simulink model "test_kalman_paper"  (R2023b)
settings: Solver=VariableStepAuto  StartTime=0.0  StopTime=30  RelTol=1e-3
values from neighbouring files (symbols this model uses):
  P0 = diag([0.01, 0.01, 0.01, 0.01, 0.01, 0.01])    [initialize_paper.m]
  Sigma = diag([0.05, 0.05, 0.05, 0.00001, 0.00001, 0.00001])    [initialize_paper.m]
  Theta = diag([0.05,0.05,0.05])    [initialize_paper.m]
libraries: simulink x2
settings Model: Creator=joaolehodey  LastModifiedBy=joaolehodey

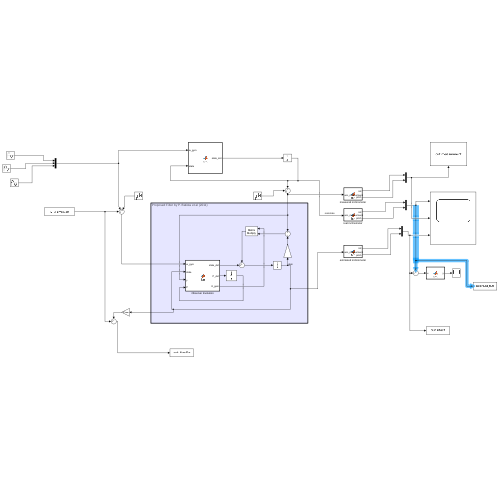
[thumbnail: Simulink's stored preview of the top-level diagram]
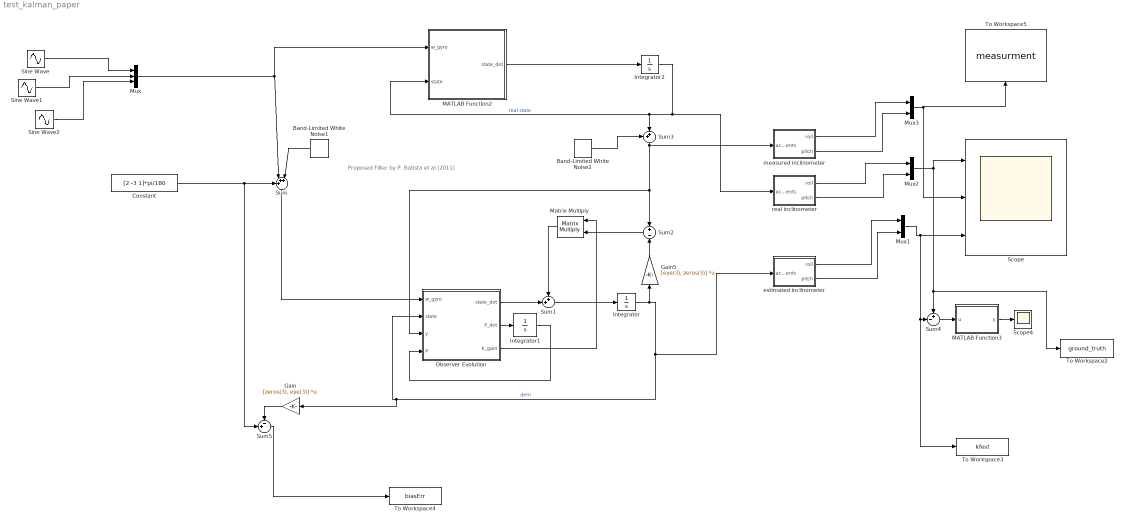
== system test_kalman_paper ==
  note: Proposed Filter by P. Batista et al (2011)
  Band-Limited White Noise1 : simulink/Sources/Band-Limited White Noise  Cov=[0.0001]*pi/180  Ts=0.01  seed=[341]  VectorParams1D=off
  Band-Limited White Noise2 : simulink/Sources/Band-Limited White Noise  Cov=[0.0001]  Ts=0.01  seed=[341]  VectorParams1D=off
  Constant : Constant  Value=[2 -3 1]*pi/180
  Gain : Gain  Gain=[zeros(3), eye(3)]  Multiplication=Matrix(K*u) (u vector)
  Gain5 : Gain  Gain=[eye(3), zeros(3)]  Multiplication=Matrix(K*u) (u vector)
  Integrator : Integrator  InitialCondition=[ 2;- 2; -9.81 ;0.0;0.0;0.0]
  Integrator1 : Integrator  InitialCondition=P0
  Integrator2 : Integrator  InitialCondition=[0, 0, -9.81]'
  MATLAB Function2 : MATLAB Function  TreatAsAtomicUnit=on
  MATLAB Function3 : MATLAB Function  TreatAsAtomicUnit=on
  Matrix Multiply : Product  Multiplication=Matrix(*)
  Mux : Mux  Inputs=3
  Mux1 : Mux  Inputs=2
  Mux2 : Mux  Inputs=2
  Mux3 : Mux  Inputs=2
  Observer Evolution : MATLAB Function  TreatAsAtomicUnit=on
  Scope : Scope  NumInputPorts=3
  Scope4 : Scope
  Sine Wave : Sin  Amplitude=-0.1  Frequency=0.5  SampleTime=0
  Sine Wave1 : Sin  Amplitude=0.1  Frequency=0.5  Phase=pi  SampleTime=0
  Sine Wave2 : Sin  Amplitude=0.1  Frequency=0.5  SampleTime=0
  Sum : Sum  Inputs=+++|
  Sum1 : Sum  Inputs=++|
  Sum2 : Sum  Inputs=+|-
  Sum3 : Sum  Inputs=++|
  Sum4 : Sum  Inputs=+-|
  Sum5 : Sum  Inputs=-+|
  To Workspace2 : ToWorkspace  VariableName=ground_truth  SaveFormat=Structure With Time  SampleTime=-1
  To Workspace3 : ToWorkspace  VariableName=kfest  SaveFormat=Structure With Time  SampleTime=-1
  To Workspace4 : ToWorkspace  VariableName=biasErr  SaveFormat=Structure With Time  SampleTime=-1
  To Workspace5 : ToWorkspace  VariableName=measurment  SaveFormat=Structure With Time  SampleTime=-1
  estimated inclinometer : MATLAB Function  TreatAsAtomicUnit=on
  measured inclinometer : MATLAB Function  TreatAsAtomicUnit=on
  real inclinometer : MATLAB Function  TreatAsAtomicUnit=on
  wires:
  Observer Evolution/1(state_dot) -> Sum1/2
  Integrator/1 -> Gain5/1, estimated inclinometer/1(acc_measurments), Gain/1, Observer Evolution/2(state)  "dem"
  Sum2/1 -> Matrix Multiply/2
  Integrator1/1 -> Observer Evolution/4(P)
  Sum1/1 -> Integrator/1
  Gain5/1 -> Sum2/2
  Observer Evolution/2(P_dot) -> Integrator1/1
  Matrix Multiply/1 -> Sum1/1
  MATLAB Function2/1(state_dot) -> Integrator2/1
  Sine Wave2/1 -> Mux/3
  Sine Wave1/1 -> Mux/2
  Sine Wave/1 -> Mux/1
  Integrator2/1 -> real inclinometer/1(acc_measurments), Sum3/2, MATLAB Function2/2(state)  "real state"
  Sum3/1 -> Observer Evolution/3(y), Sum2/1, measured inclinometer/1(acc_measurments)
  Mux/1 -> MATLAB Function2/1(w_gyro), Sum/2
  estimated inclinometer/1(roll) -> Mux1/1
  estimated inclinometer/2(pitch) -> Mux1/2
  real inclinometer/1(roll) -> Mux2/1
  real inclinometer/2(pitch) -> Mux2/2
  Constant/1 -> Sum/1, Sum5/2
  Sum/1 -> Observer Evolution/1(w_gyro)
  Band-Limited White Noise2/1 -> Sum3/1
  Band-Limited White Noise1/1 -> Sum/3
  Observer Evolution/3(K_gain) -> Matrix Multiply/1
  Mux1/1 -> Scope/3, To Workspace3/1, Sum4/2
  Mux2/1 -> Scope/1, To Workspace2/1, Sum4/1
  Sum4/1 -> MATLAB Function3/1(u)
  MATLAB Function3/1(y) -> Scope4/1
  Gain/1 -> Sum5/1
  Sum5/1 -> To Workspace4/1
  measured inclinometer/1(roll) -> Mux3/1
  measured inclinometer/2(pitch) -> Mux3/2
  Mux3/1 -> To Workspace5/1, Scope/2

== matlab function test_kalman_paper/Observer Evolution ==
  data: w_gyro input; state input; y input; state_dot output; P_dot output; P input; Sigma parameter; Theta parameter; K_gain output
function [state_dot, P_dot, K_gain]= fcn(w_gyro, state,y,P, Sigma, Theta)

%y = state(1:3);
%bias = state(4:6);

C = [eye(3), zeros(3)];


skew_gyro = [0 -w_gyro(3)  w_gyro(2) ; w_gyro(3) 0 -w_gyro(1) ; -w_gyro(2) w_gyro(1) 0 ];

skew_att = [0 -y(3) y(2) ; y(3) 0 -y(1) ; -y(2) y(1) 0 ];

% build time varying matrix A
A = [-skew_gyro, -skew_att; zeros(3), zeros(3)];

state_dot = A*state;


P_dot = A*P + P*A' + Sigma - P*C'*inv(Theta)*C*P; 
K_gain = P*C'*inv(Theta); %#ok<*MINV>

== matlab function test_kalman_paper/MATLAB Function2 ==
  data: w_gyro input; state input; state_dot output
function state_dot = fcn(w_gyro, state)

%attitude = state(1:3);
%bias = state(4:6);

skew_gyro = [0 -w_gyro(3) w_gyro(2) ; w_gyro(3) 0 -w_gyro(1) ; -w_gyro(2) w_gyro(1) 0 ];
%A = [-skew_gyro];

state_dot = -skew_gyro*state;

== matlab function test_kalman_paper/measured inclinometer ==
  data: acc_measurments input; roll output; pitch output
function [roll, pitch] = fcn(acc_measurments)
ax = acc_measurments(1);
ay = acc_measurments(2);
az = acc_measurments(3);

ag = sqrt(ax*ax + ay*ay + az*az);
if ag == 0
    pitch = 0;
    roll = 0;
    return
end

roll = atan(ay/az);
pitch = asin(ax/ag);

== matlab function test_kalman_paper/real inclinometer ==
  data: acc_measurments input; roll output; pitch output
function [roll, pitch] = fcn(acc_measurments)
ax = acc_measurments(1);
ay = acc_measurments(2);
az = acc_measurments(3);

ag = sqrt(ax*ax + ay*ay + az*az);
if ag == 0
    pitch = 0;
    roll = 0;
    return
end

roll = atan(ay/az);
pitch = asin(ax/ag);

== matlab function test_kalman_paper/estimated inclinometer ==
  data: acc_measurments input; roll output; pitch output
function [roll, pitch] = fcn(acc_measurments)
ax = acc_measurments(1);
ay = acc_measurments(2);
az = acc_measurments(3);

ag = sqrt(ax*ax + ay*ay + az*az);
if ag == 0
    pitch = 0;
    roll = 0;
    return
end

roll = atan(ay/az);
pitch = asin(ax/ag);

== matlab function test_kalman_paper/MATLAB Function3 ==
  data: u input; y output
function y = fcn(u)

y = norm(u);
